simulink model "roll_loop"  (R2016a)
settings: Solver=VariableStepAuto  StartTime=0.0  StopTime=20.0  RelTol=1e-3
values from neighbouring files (symbols this model uses):
  a_phi1 = 16.2447    [tune_roll.m]
  a_phi2 = 128.0716    [tune_roll.m]
  roll_kd = (2*zeta_roll*wn_roll - a_phi1)/a_phi2    [tune_roll.m]
  roll_ki = 0.2    [tune_roll.m]
  roll_kp = wn_roll^2/a_phi2    [tune_roll.m]
settings Model: Creator=andreanv  LastModifiedBy=andreanv

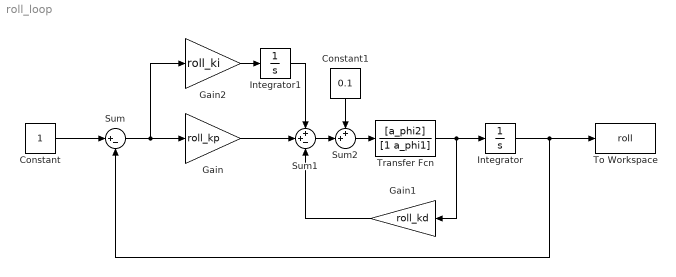
== system roll_loop ==
  Constant : Constant
  Constant1 : Constant  Value=0.1
  Gain : Gain  Gain=roll_kp
  Gain1 : Gain  Gain=roll_kd
  Gain2 : Gain  Gain=roll_ki
  Integrator : Integrator
  Integrator1 : Integrator
  Sum : Sum  Inputs=|+-
  Sum1 : Sum  Inputs=++-
  Sum2 : Sum  Inputs=++|
  To Workspace : ToWorkspace  VariableName=roll  SaveFormat=Timeseries  SampleTime=-1
  Transfer Fcn : TransferFcn  Numerator=[a_phi2]  Denominator=[1 a_phi1]
  wires:
  Constant/1 -> Sum/1
  Sum/1 -> Gain2/1, Gain/1
  Transfer Fcn/1 -> Gain1/1, Integrator/1
  Integrator/1 -> Sum/2, To Workspace/1
  Sum1/1 -> Sum2/2
  Sum2/1 -> Transfer Fcn/1
  Constant1/1 -> Sum2/1
  Gain2/1 -> Integrator1/1
  Integrator1/1 -> Sum1/1
  Gain1/1 -> Sum1/3
  Gain/1 -> Sum1/2
